simulink model "BLDCMODELTOTALNEURON"  (R2020a)
settings: Solver=ode45  StartTime=0.0  StopTime=2  RelTol=1e-3  EnableMultiTasking=on
InitFcn:
  | clc;
StopFcn:
  | clc;
undefined symbols (not defined in the file): sigbuilder_block, Ts
libraries: neural x55, fl_lib x14, nesl_utility x14, simulink x7, spsIGBTDiodeLib x6, spsVoltageMeasurementLib x3, powerlib_extras x1, spsControlledVoltageSourceLib x1, spsGroundLib x1, spsThreePhaseVIMeasurementLib x1, spspowerguiLib x1
(part 3 of 3)

== system BLDCMODELTOTALNEURON/Function Fitting Neural Network/Layer 2/LW{2,1} ==
  "ad{2,1}" : Inport  PortDimensions=50
      mask Display: e = 0.06;c1 = [120 230 180]/255;c2 = ([120 230 180]+0)/(256+128);c3 = ([120 230 180]+128)/(256+128);patch([0 1 1 0],[0 0 1 1],c1);patch([0 1 1 1-e 1-e 0+e],[0 0 1 1-e 0+e 0+e],c2);patch([0 0 1 1-e 0+e 0+e],[0 1 1 1-e 1-e 0+e],c3);plot([0 1 1 0 0],[0 0 1 1 0]);
  "IW{2,1}(1,:)'" : Constant  Value=[3.816339594498053156002015384729020297527313232421875;-6.2711019201511017939765224582515656948089599609375;-3.245160958716878152330309603712521493434906005859375;3.685270600204774371633220653166063129901885986328125;-1.326796308424502246481324618798680603504180908203125;2.733083901954909133991122871520929038524627685546875;-5.90809916797024126111637087888084352016448974609375;10.9047920138566905023935760254971683025360107421875;-4.0861125636681858708243453293107450008392333984375;-7.255053299137120603745643165893852710723876953125;-5.1841946464846841990947723388671875;-2.018556593641415819462281433516182005405426025390625;1.684383772262440626121815512306056916713714599609375;5.00530768226195732495398260653018951416015625;6.5633756370814158032089835614897310733795166015625;-9.0024297092309968348899928969331085681915283203125;-10.27245155582406965777408913709223270416259765625;-8.0422217956168964292373857460916042327880859375;8.5644854944461510370956602855585515499114990234375;-2.6703466596190761350726461387239396572113037109375;-4.3287991274016963672011115704663097858428955078125;3.574915184853874716708332925918512046337127685546875;12.10830210180603927483389270491898059844970703125;-3.55930499454568671779952637734822928905487060546875;4.34172912385168530136070330627262592315673828125;9.688352177251562835635922965593636035919189453125;1.778793094836221388987951286253519356250762939453125;-8.2989540526607132875369643443264067173004150390625;5.11609954451892345872465739375911653041839599609375;-5.44599034819631899750902448431588709354400634765625;-5.9859465865708418874646667973138391971588134765625;4.927294138573341086839718627743422985076904296875;0.345490416766692065575483638895093463361263275146484375;6.894781120094325643776755896396934986114501953125;-5.45012226062890103861491297720931470394134521484375;2.795447522217527680510329446406103670597076416015625;-4.91773660022124570190271697356365621089935302734375;-10.8622692002469278804710484109818935394287109375;-4.72133195210023881571714809979312121868133544921875;3.078436937982767407362416633986867964267730712890625;1.077647019535872718876134968013502657413482666015625;5.20763759755854405142372343107126653194427490234375;5.39255440552966280876034943503327667713165283203125;-2.175358250171595120292522551608271896839141845703125;-3.2009547273914424891927410499192774295806884765625;-8.9500381407923352838906794204376637935638427734375;-4.7711598908392289786206674762070178985595703125;3.32579957605036025114486619713716208934783935546875;6.1192084237935713275646776310168206691741943359375;-2.723355638124754563023088849149644374847412109375]
      mask Display: e = 0.06;c1 = [120 150 230]/255;c2 = ([120 150 230]+0)/383;c3 = ([120 150 230]+128)/383;patch([0 1 1 0],[0 0 1 1],c1);patch([0 1 1 1-e 1-e 0+e],[0 0 1 1-e 0+e 0+e],c2);patch([0 0 1 1-e 0+e 0+e],[0 1 1 1-e 1-e 0+e],c3);plot([0 1 1 0 0],[0 0 1 1 0]);disp('weights');
  Mux : Mux  Inputs=1
      mask Display: e = 0.06;c1 = [120 150 230]/255;c2 = ([120 150 230]+0)/383;c3 = ([120 150 230]+128)/383;patch([0 1 1 0],[0 0 1 1],c1);patch([0 1 1 1-e 1-e 0+e],[0 0 1 1-e 0+e 0+e],c2);patch([0 0 1 1-e 0+e 0+e],[0 1 1 1-e 1-e 0+e],c3);plot([0 1 1 0 0],[0 0 1 1 0]);disp('Mux');
  dotprod1 : neural/Weight Functions/dotprod
  "lz{2,1}" : Outport
      mask Display: e = 0.06;c1 = [120 230 180]/255;c2 = ([120 230 180]+0)/(256+128);c3 = ([120 230 180]+128)/(256+128);patch([0 1 1 0],[0 0 1 1],c1);patch([0 1 1 1-e 1-e 0+e],[0 0 1 1-e 0+e 0+e],c2);patch([0 0 1 1-e 0+e 0+e],[0 1 1 1-e 1-e 0+e],c3);plot([0 1 1 0 0],[0 0 1 1 0]);
  wires:
  "IW{2,1}(1,:)'"/1 -> dotprod1/1
  "ad{2,1}"/1 -> dotprod1/2
  dotprod1/1 -> Mux/1
  Mux/1 -> "lz{2,1}"/1

== system BLDCMODELTOTALNEURON/BLDC Model/current generater/state equations/State Ib ==
  Vab,Vbc : Inport
  Eabc : Inport  Port=2
  Fcn : Fcn  Expr=-u(1)+u(2)+u(3)-2*u(4)+u(5)-3*2.8750*u(6)
  Gain2 : Gain  Gain=1/(3*.0085)  SaturateOnIntegerOverflow=on  OutDataTypeStr=Inherit: Same as input  ParamDataTypeStr=Inherit: Same as input
  Mux : Mux  Inputs=3
  "s " : Integrator
  i : Outport
  wires:
  Gain2/1 -> "s "/1
  Vab,Vbc/1 -> Mux/1
  Eabc/1 -> Mux/2
  Mux/1 -> Fcn/1
  Fcn/1 -> Gain2/1
  "s "/1 -> Mux/3, i/1

== system BLDCMODELTOTALNEURON/BLDC Model/current generater/state equations/state Ia ==
  Vab,Vbc : Inport
  Eabc : Inport  Port=2
  Fcn : Fcn  Expr=2*u(1)+u(2)-2*u(3)+u(4)+u(5)-3*2.8750*u(6)
  Gain2 : Gain  Gain=1/(3*.0085)  SaturateOnIntegerOverflow=on  OutDataTypeStr=Inherit: Same as input  ParamDataTypeStr=Inherit: Same as input
  Mux : Mux  Inputs=3
  "s " : Integrator
  i : Outport
  wires:
  "s "/1 -> Mux/3, i/1
  Fcn/1 -> Gain2/1
  Mux/1 -> Fcn/1
  Eabc/1 -> Mux/2
  Vab,Vbc/1 -> Mux/1
  Gain2/1 -> "s "/1

== system BLDCMODELTOTALNEURON/BLDC Model/emf generation/Phase a/cos (u(1)) ==
  In1 : Inport
  Fcn : Fcn  Expr=cos(u(1))
  Saturation : Saturate  UpperLimit=0.8  LowerLimit=-0.8
  Out1 : Outport
  wires:
  In1/1 -> Fcn/1
  Fcn/1 -> Saturation/1
  Saturation/1 -> Out1/1

== system BLDCMODELTOTALNEURON/BLDC Model/emf generation/Phase b/cos (u(1)) ==
  In1 : Inport
  Fcn : Fcn  Expr=cos(u(1)-2*pi/3)
  Saturation : Saturate  UpperLimit=0.8  LowerLimit=-0.8
  Out1 : Outport
  wires:
  In1/1 -> Fcn/1
  Fcn/1 -> Saturation/1
  Saturation/1 -> Out1/1

== system BLDCMODELTOTALNEURON/BLDC Model/emf generation/Phase c/cos (u(1)) ==
  In1 : Inport
  Fcn1 : Fcn  Expr=cos(u(1)+2*pi/3)
  Saturation : Saturate  UpperLimit=0.8  LowerLimit=-0.8
  Out1 : Outport
  wires:
  In1/1 -> Fcn1/1
  Fcn1/1 -> Saturation/1
  Saturation/1 -> Out1/1

== matlab function BLDCMODELTOTALNEURON/MATLAB Function1 ==
  data: Normal output; U input; T1 output; T2 output; T3 output; T4 output; T5 output; T6 output
function [Normal,T1, T2, T3, T4, T5, T6] = decoder(U)
    % Initialisation des sorties
    Normal=0;
    T1 = 0;
    T2 = 0;
    T3 = 0;
    T4 = 0;
    T5 = 0;
    T6 = 0;

    % Décodeur en fonction de l'entrée U
    switch U
        case 1
            Normal=1;
        case 2
            T1 = 1;
        case 3
            T2 = 1;
        case 4
            T3 = 1;
        case 5
            T4 = 1;
        case 6
            T5 = 1;
        case 7
            T6 = 1;
        case 8
            T1 = 1;
            T2 = 1;
        case 9
            T3 = 1;
            T4 = 1;
        case 10
            T5 = 1;
            T6 = 1;
        case 11
            T2 = 1;
            T3 = 1;
        case 12
            T3 = 1;
            T5 = 1;
        case 13
            T4 = 1;
            T6 = 1;
        case 14
            T2 = 1;
            T4 = 1;
        case 15
            T5 = 1;
        case 16
            T1 = 1;
            T5 = 1;
        case 17
            T4 = 1;
            T5 = 1;
            T6 = 1;
        case 18
            T1 = 1;
            T2 = 1;
            T3 = 1;
        case 19
            T2 = 1;
            T4 = 1;
            T6 = 1;
        
    end
end

== matlab function BLDCMODELTOTALNEURON/MATLAB Function2 ==
  data: Ia input; Ia_mean output; Ib input; Ic input; Ib_mean output; Ic_mean output; atanBA output; atanCA output; atanAC output; atanBC output; atanAB output; atanCB output
function [Ia_mean, Ib_mean, Ic_mean, atanBA, atanCA, atanAC, atanBC, atanAB, atanCB] = computeRunningMeans(Ia, Ib, Ic)
% This function computes the running mean of the currents Ia, Ib, and Ic

% Persistent variables to accumulate the sum and count
persistent sum_Ia sum_Ib sum_Ic count;

% Initialize persistent variables on the first run
if isempty(sum_Ia)
    sum_Ia = 0;
    sum_Ib = 0;
    sum_Ic = 0;
    count = 0;
end

% Accumulate the currents
sum_Ia = sum_Ia + Ia;
sum_Ib = sum_Ib + Ib;
sum_Ic = sum_Ic + Ic;

% Increment the count
count = count + 1;

% Compute the running mean
Ia_mean = sum_Ia / count;
Ib_mean = sum_Ib / count;
Ic_mean = sum_Ic / count;

% Compute the arctangents of the mean ratios and convert to degrees
atanBA = atan2d(Ib_mean, Ia_mean);
atanCA = atan2d(Ic_mean, Ia_mean);
atanAC = atan2d(Ia_mean, Ic_mean);
atanBC = atan2d(Ib_mean, Ic_mean);
atanAB = atan2d(Ia_mean, Ib_mean);
atanCB = atan2d(Ic_mean, Ib_mean);

end

== matlab function BLDCMODELTOTALNEURON/MATLAB Function3 ==
  data: valeur input; entierPlusProche output
function entierPlusProche = fcn(valeur)
    entierPlusProche = round(valeur);  % Arrondit la valeur à l'entier le plus proche
end
